simulink model "crane_sim"  (Simulink 8.3)
settings: Solver=ode45  StartTime=0.0  StopTime=200  RelTol=1e-3
undefined symbols (not defined in the file or in its folder): drawGantryCrane, P
libraries: cstblocks x2
settings Model: Creator=beard  LastModifiedBy=jhl48
settings OptimizationCC: ExpressionDepthLimit=2147483647  InitFltsAndDblsToZero=on
settings DebuggingCC: FcnCallInpInsideContextMsg=UseLocalSettings

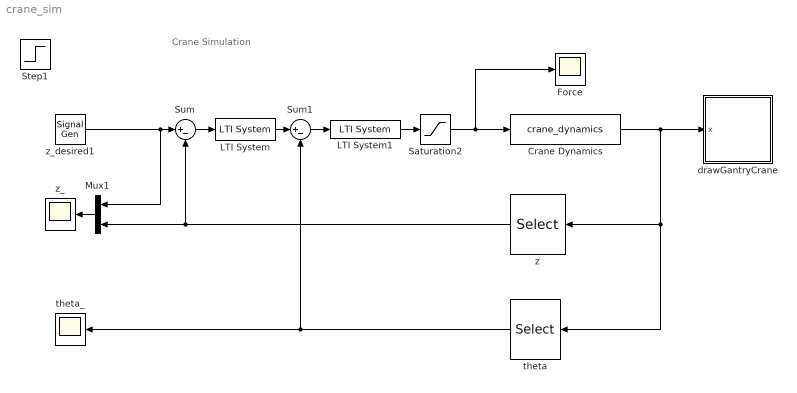
== system crane_sim ==
  note: Crane Simulation
  Crane Dynamics : S-Function  FunctionName=crane_dynamics  Parameters=P  EnableBusSupport=off
  Force : Scope
      settings: TimeRange=100  YMin=-1000  YMax=1250
  LTI System : cstblocks/LTI System  sys=c_outer  IC=[]
  LTI System1 : cstblocks/LTI System  sys=c_inner  IC=[]
  Mux1 : Mux  Inputs=2
  Saturation2 : Saturate  UpperLimit=P.F_max  LowerLimit=-P.F_max
  Step1 : Step  Time=20  After=7  SampleTime=0
  Sum : Sum  Inputs=|+-
  Sum1 : Sum  Inputs=|+-
  drawGantryCrane : Subsystem
      mask init:
      | bar = 20;
      | crane = [5 3];
      | L1 = 10;
      | R1 = 1;
      mask Display: image(imread('tv.jpg'))
  theta : Selector  InputPortWidth=4  Indices=[4]
  theta_ : Scope
      settings: TimeRange=100  YMin=-0.2  YMax=0.2
  z : Selector  InputPortWidth=4  Indices=[3]
  z_ : Scope
      settings: TimeRange=100  YMin=-8  YMax=7  SaveName=ScopeData2
  z_desired1 : SignalGenerator  WaveForm=square  Amplitude=7  Frequency=.01
  wires:
  Crane Dynamics/1 -> theta/1, z/1, drawGantryCrane/1(x)
  Mux1/1 -> z_/1
  Saturation2/1 -> Crane Dynamics/1, Force/1
  z_desired1/1 -> Sum/1, Mux1/1
  z/1 -> Sum/2, Mux1/2
  theta/1 -> Sum1/2, theta_/1
  Sum/1 -> LTI System/1
  LTI System/1 -> Sum1/1
  Sum1/1 -> LTI System1/1
  LTI System1/1 -> Saturation2/1

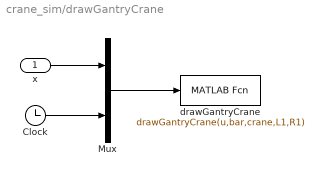
== system crane_sim/drawGantryCrane ==
  x : Inport
  Clock : Clock
  Mux : Mux  Inputs=2
  drawGantryCrane : MATLABFcn  MATLABFcn=drawGantryCrane(u,bar,crane,L1,R1)  OutputDimensions=0  SampleTime=0.1
  wires:
  Mux/1 -> drawGantryCrane/1
  x/1 -> Mux/1
  Clock/1 -> Mux/2
